simulink subsystem "shaping"  (R2024b)
settings: Solver=VariableStepAuto  StartTime=0.0  StopTime=10.0  RelTol=1e-3
model mask{c_srrc_coef=0, c_inter_1_coef=0, c_inter_2_coef=0}
  mask prompts: c_srrc_coef "Interpolator SRRC  stage coefficients"; c_inter_1_coef "Interpolator 1 coefficients"; c_inter_2_coef "Interpolator 2 coefficients"
values from neighbouring files (symbols this model uses):
  c_srrc_coef = jsonData.shaping.c_srrc_coef    [seq.m]
libraries: hdlsllib x10, dsphdlfiltering2 x3
settings Model: Creator=usradmin  LastModifiedBy=jose.sanchez
settings RTWCC: GPUComputeCapability=3.5

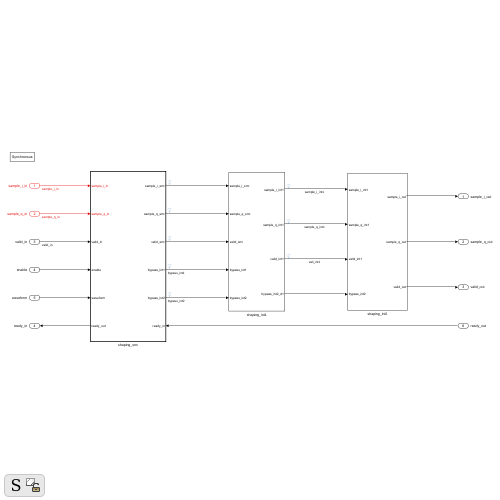
[thumbnail: Simulink's stored preview of the top-level diagram]
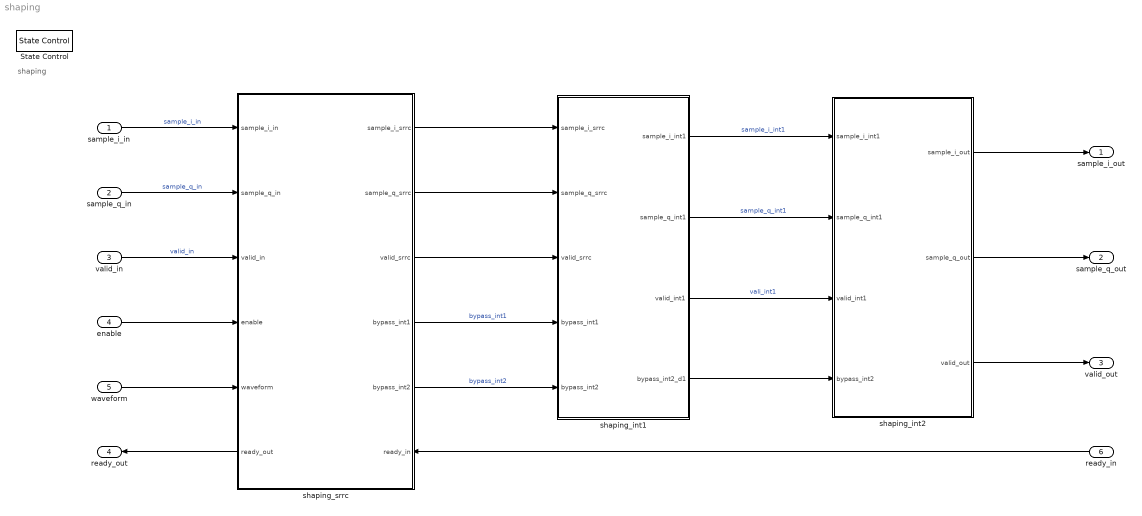
== system shaping ==
  note: shaping
  sample_i_in : Inport  OutDataTypeStr=fixdt(1,16,15)
  sample_q_in : Inport  Port=2  OutDataTypeStr=fixdt(1,16,15)
  valid_in : Inport  Port=3  OutDataTypeStr=boolean
  enable : Inport  Port=4  OutDataTypeStr=boolean
  waveform : Inport  Port=5  OutMin=[0]  OutMax=[3]  OutDataTypeStr=fixdt(0,2)
  ready_in : Inport  Port=6  OutDataTypeStr=boolean
  State Control : StateControl  StateControl=Synchronous
  shaping_int1 : Subsystem
  shaping_int2 : Subsystem
  shaping_srrc : Subsystem
      settings: PortSchema="{\"entries\":[{\"content\":{\"sides\":[{\"content\":{\"connectorIds\":[\"In1\",\"In2\",\"In3\",\"In4\",\"In5\",\"Out6\"]},\"type\":\"ConnectorPlacement.EquallySpacedRectSide\",\"uuid\":\"d1664757-8441-4e5c-b538-f30b5bedf7ee\"},{\"content\":{\"connectorIds\":[\"Out1\",\"Out2\",\"Out3\",\"Out4\",\"Out5\",\"In6\"],\"side\":\"RIGHT\"},\"type\":\"ConnectorPlacement.EquallySpacedRectSide\",\"uuid\":\"660e1ba2-a444-4ece-b784-c0538aecc110\"},{\"content\":{\"side\":\"TOP\"},\"type\":\"ConnectorPlacement.EquallySpacedRectSide\",\"uuid\":\"adc6c3d6-bacf-46d3-9822-3cabe58d745e\"}]},\"type\":\"ConnectorPlacement.EquallySpacedConnector\",\"uuid\":\"1ec29908-4970-4c2d-ab54-8f6747339545\"}],\"packageUris\":[\"http://schema.mathworks.com/mf0/Connector/R2020b\"],\"version\":\"1.0\"}"
  sample_i_out : Outport  OutDataTypeStr=fixdt(1,16,14)
  sample_q_out : Outport  Port=2  OutDataTypeStr=fixdt(1,16,14)
  valid_out : Outport  Port=3  OutDataTypeStr=boolean
  ready_out : Outport  Port=4  OutDataTypeStr=boolean
  wires:
  sample_i_in/1 -> shaping_srrc/1(sample_i_in)  "sample_i_in"
  sample_q_in/1 -> shaping_srrc/2(sample_q_in)  "sample_q_in"
  valid_in/1 -> shaping_srrc/3(valid_in)  "valid_in"
  shaping_srrc/6(ready_out) -> ready_out/1
  enable/1 -> shaping_srrc/4(enable)
  waveform/1 -> shaping_srrc/5(waveform)
  shaping_srrc/1(sample_i_srrc) -> shaping_int1/1(sample_i_srrc)
  shaping_srrc/2(sample_q_srrc) -> shaping_int1/2(sample_q_srrc)
  shaping_srrc/3(valid_srrc) -> shaping_int1/3(valid_srrc)
  shaping_srrc/4(bypass_int1) -> shaping_int1/4(bypass_int1)  "bypass_int1"
  shaping_int1/1(sample_i_int1) -> shaping_int2/1(sample_i_int1)  "sample_i_int1"
  shaping_int1/2(sample_q_int1) -> shaping_int2/2(sample_q_int1)  "sample_q_int1"
  shaping_int1/3(valid_int1) -> shaping_int2/3(valid_int1)  "vali_int1"
  shaping_int2/1(sample_i_out) -> sample_i_out/1
  shaping_int2/2(sample_q_out) -> sample_q_out/1
  shaping_int2/3(valid_out) -> valid_out/1
  ready_in/1 -> shaping_srrc/6(ready_in)
  shaping_srrc/5(bypass_int2) -> shaping_int1/5(bypass_int2)  "bypass_int2"
  shaping_int1/4(bypass_int2_d1) -> shaping_int2/4(bypass_int2)

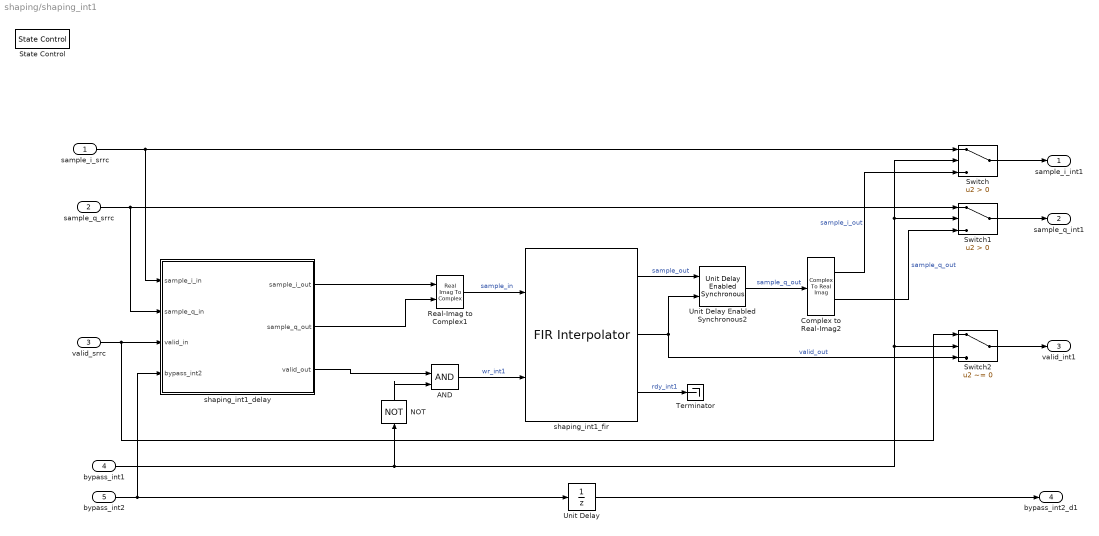
== system shaping/shaping_int1 ==
  sample_i_srrc : Inport
  sample_q_srrc : Inport  Port=2
  valid_srrc : Inport  Port=3
  bypass_int1 : Inport  Port=4
  bypass_int2 : Inport  Port=5
  AND : Logic  IconShape=distinctive  AllPortsSameDT=off  OutDataTypeStr=boolean
  Complex to Real-Imag2 : ComplexToRealImag
  NOT : Logic  Operator=NOT  IconShape=distinctive  AllPortsSameDT=off  OutDataTypeStr=boolean
  Real-Imag to Complex1 : RealImagToComplex
  State Control : StateControl  StateControl=Synchronous
  Switch : Switch  Criteria=u2 > Threshold  SaturateOnIntegerOverflow=off  InputSameDT=off
  Switch1 : Switch  Criteria=u2 > Threshold  SaturateOnIntegerOverflow=off  InputSameDT=off
  Switch2 : Switch  Criteria=u2 ~= 0  SaturateOnIntegerOverflow=off  InputSameDT=off
  Terminator : Terminator
  Unit Delay : UnitDelay  SampleTime=-1  HasFrameUpgradeWarning=on
  Unit Delay Enabled Synchronous2 : hdlsllib/Discrete/Unit Delay Enabled Synchronous  InitialCondition=0.0  SampleTime=-1
  shaping_int1_delay : Subsystem
  shaping_int1_fir : dsphdlfiltering2/FIR Interpolator  Numerator=c_inter_1_coef  FilterStructure=Direct form systolic  InterpolationFactor=2  NumCycles=2  OptimizeSymmCoeff=on  SimulateUsing=Code generation  roundingMode=Floor  overflowMode=off  CoefficientsDataTypeStr=fixdt(1,16,15)  OutputDataTypeStr=fixdt(1,16,14)  ResetInputPort=off  HDLGlobalReset=on
  sample_i_int1 : Outport
  sample_q_int1 : Outport  Port=2
  valid_int1 : Outport  Port=3
  bypass_int2_d1 : Outport  Port=4
  wires:
  Unit Delay/1 -> bypass_int2_d1/1
  bypass_int2/1 -> Unit Delay/1, shaping_int1_delay/4(bypass_int2)
  valid_srrc/1 -> shaping_int1_delay/3(valid_in), Switch2/1
  sample_q_srrc/1 -> shaping_int1_delay/2(sample_q_in), Switch1/1
  sample_i_srrc/1 -> Switch/1, shaping_int1_delay/1(sample_i_in)
  shaping_int1_fir/3 -> Terminator/1  "rdy_int1"
  Switch2/1 -> valid_int1/1
  Real-Imag to Complex1/1 -> shaping_int1_fir/1  "sample_in"
  shaping_int1_delay/2(sample_q_out) -> Real-Imag to Complex1/2
  bypass_int1/1 -> NOT/1, Switch2/2, Switch1/2, Switch/2
  shaping_int1_delay/3(valid_out) -> AND/1
  Switch/1 -> sample_i_int1/1
  AND/1 -> shaping_int1_fir/2  "wr_int1"
  Complex to Real-Imag2/2 -> Switch1/3  "sample_q_out"
  Switch1/1 -> sample_q_int1/1
  shaping_int1_delay/1(sample_i_out) -> Real-Imag to Complex1/1
  Unit Delay Enabled Synchronous2/1 -> Complex to Real-Imag2/1  "sample_q_out"
  shaping_int1_fir/2 -> Unit Delay Enabled Synchronous2/2, Switch2/3  "valid_out"
  shaping_int1_fir/1 -> Unit Delay Enabled Synchronous2/1  "sample_out"
  NOT/1 -> AND/2
  Complex to Real-Imag2/1 -> Switch/3  "sample_i_out"

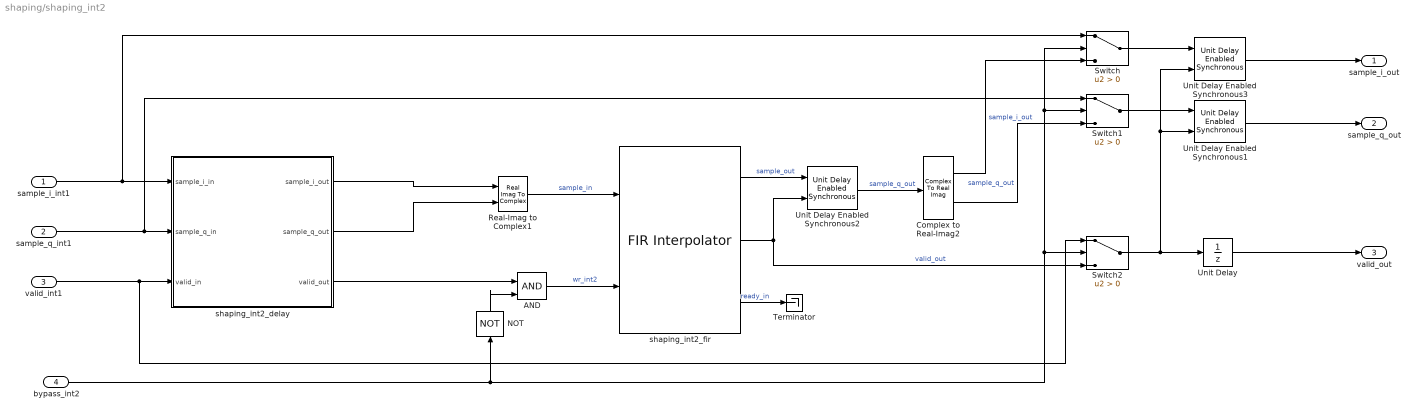
== system shaping/shaping_int2 ==
  sample_i_int1 : Inport
  sample_q_int1 : Inport  Port=2
  valid_int1 : Inport  Port=3
  bypass_int2 : Inport  Port=4
  AND : Logic  IconShape=distinctive  AllPortsSameDT=off  OutDataTypeStr=boolean
  Complex to Real-Imag2 : ComplexToRealImag
  NOT : Logic  Operator=NOT  IconShape=distinctive  AllPortsSameDT=off  OutDataTypeStr=boolean
  Real-Imag to Complex1 : RealImagToComplex
  Switch : Switch  Criteria=u2 > Threshold  SaturateOnIntegerOverflow=off  InputSameDT=off
  Switch1 : Switch  Criteria=u2 > Threshold  SaturateOnIntegerOverflow=off  InputSameDT=off
  Switch2 : Switch  Criteria=u2 > Threshold  SaturateOnIntegerOverflow=off  InputSameDT=off
  Terminator : Terminator
  Unit Delay : UnitDelay  SampleTime=-1  HasFrameUpgradeWarning=on
  Unit Delay Enabled Synchronous1 : hdlsllib/Discrete/Unit Delay Enabled Synchronous  InitialCondition=0.0  SampleTime=-1
  Unit Delay Enabled Synchronous2 : hdlsllib/Discrete/Unit Delay Enabled Synchronous  InitialCondition=0.0  SampleTime=-1
  Unit Delay Enabled Synchronous3 : hdlsllib/Discrete/Unit Delay Enabled Synchronous  InitialCondition=0.0  SampleTime=-1
  shaping_int2_delay : Subsystem
  shaping_int2_fir : dsphdlfiltering2/FIR Interpolator  Numerator=c_inter_2_coef  FilterStructure=Direct form systolic  InterpolationFactor=2  NumCycles=2  OptimizeSymmCoeff=on  SimulateUsing=Code generation  roundingMode=Floor  overflowMode=off  CoefficientsDataTypeStr=fixdt(1,16,15)  OutputDataTypeStr=fixdt(1,16,14)  ResetInputPort=off  HDLGlobalReset=on
  sample_i_out : Outport
  sample_q_out : Outport  Port=2
  valid_out : Outport  Port=3
  wires:
  valid_int1/1 -> shaping_int2_delay/3(valid_in), Switch2/1
  sample_q_int1/1 -> shaping_int2_delay/2(sample_q_in), Switch1/1
  sample_i_int1/1 -> shaping_int2_delay/1(sample_i_in), Switch/1
  Unit Delay/1 -> valid_out/1
  Switch/1 -> Unit Delay Enabled Synchronous3/1
  Switch1/1 -> Unit Delay Enabled Synchronous1/1
  Complex to Real-Imag2/1 -> Switch/3  "sample_i_out"
  NOT/1 -> AND/2
  shaping_int2_fir/1 -> Unit Delay Enabled Synchronous2/1  "sample_out"
  shaping_int2_fir/2 -> Unit Delay Enabled Synchronous2/2, Switch2/3  "valid_out"
  Unit Delay Enabled Synchronous2/1 -> Complex to Real-Imag2/1  "sample_q_out"
  shaping_int2_delay/1(sample_i_out) -> Real-Imag to Complex1/1
  Unit Delay Enabled Synchronous1/1 -> sample_q_out/1
  shaping_int2_fir/3 -> Terminator/1  "ready_in"
  Complex to Real-Imag2/2 -> Switch1/3  "sample_q_out"
  AND/1 -> shaping_int2_fir/2  "wr_int2"
  Unit Delay Enabled Synchronous3/1 -> sample_i_out/1
  shaping_int2_delay/3(valid_out) -> AND/1
  bypass_int2/1 -> NOT/1, Switch1/2, Switch/2, Switch2/2
  shaping_int2_delay/2(sample_q_out) -> Real-Imag to Complex1/2
  Real-Imag to Complex1/1 -> shaping_int2_fir/1  "sample_in"
  Switch2/1 -> Unit Delay/1, Unit Delay Enabled Synchronous3/2, Unit Delay Enabled Synchronous1/2

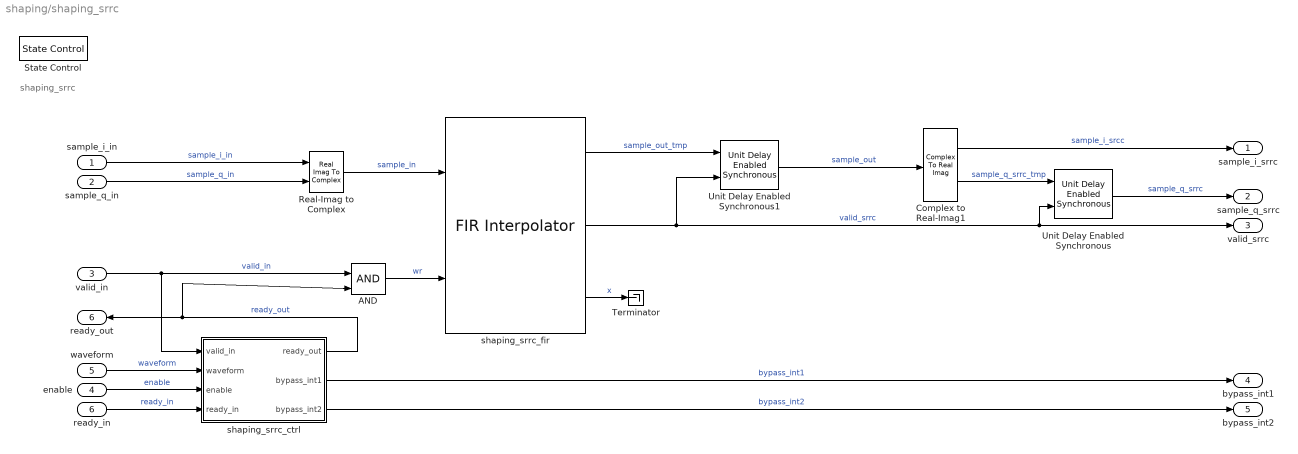
== system shaping/shaping_srrc ==
  note: shaping_srrc
  sample_i_in : Inport  OutDataTypeStr=fixdt(1,16,15)
  sample_q_in : Inport  Port=2  OutDataTypeStr=fixdt(1,16,15)
  valid_in : Inport  Port=3  OutDataTypeStr=boolean
  enable : Inport  Port=4  OutDataTypeStr=boolean
  waveform : Inport  Port=5  OutMin=[0]  OutMax=[3]  OutDataTypeStr=fixdt(0,2)
  ready_in : Inport  Port=6  OutDataTypeStr=boolean
  AND : Logic  IconShape=distinctive  AllPortsSameDT=off  OutDataTypeStr=boolean
  Complex to Real-Imag1 : ComplexToRealImag
  Real-Imag to Complex : RealImagToComplex
  State Control : StateControl  StateControl=Synchronous
  Terminator : Terminator
  Unit Delay Enabled Synchronous : hdlsllib/Discrete/Unit Delay Enabled Synchronous  InitialCondition=0.0  SampleTime=-1
  Unit Delay Enabled Synchronous1 : hdlsllib/Discrete/Unit Delay Enabled Synchronous  InitialCondition=0.0  SampleTime=-1
  shaping_srrc_ctrl : MATLAB Function  TreatAsAtomicUnit=on
  shaping_srrc_fir : dsphdlfiltering2/FIR Interpolator  Numerator=c_srrc_coef  FilterStructure=Direct form systolic  InterpolationFactor=2  NumCycles=2  OptimizeSymmCoeff=on  SimulateUsing=Code generation  roundingMode=Floor  overflowMode=off  CoefficientsDataTypeStr=fixdt(1,16,15)  OutputDataTypeStr=fixdt(1,16,14)  ResetInputPort=off  HDLGlobalReset=on
  sample_i_srrc : Outport
  sample_q_srrc : Outport  Port=2
  valid_srrc : Outport  Port=3  OutDataTypeStr=boolean
  bypass_int1 : Outport  Port=4  OutDataTypeStr=boolean
  bypass_int2 : Outport  Port=5  OutDataTypeStr=boolean
  ready_out : Outport  Port=6  OutDataTypeStr=boolean
  wires:
  ready_in/1 -> shaping_srrc_ctrl/4(ready_in)  "ready_in"
  shaping_srrc_fir/3 -> Terminator/1  "x"
  shaping_srrc_ctrl/3(bypass_int2) -> bypass_int2/1  "bypass_int2"
  shaping_srrc_ctrl/2(bypass_int1) -> bypass_int1/1  "bypass_int1"
  Unit Delay Enabled Synchronous/1 -> sample_q_srrc/1  "sample_q_srrc"
  valid_in/1 -> shaping_srrc_ctrl/1(valid_in), AND/1  "valid_in"
  sample_i_in/1 -> Real-Imag to Complex/1  "sample_i_in"
  enable/1 -> shaping_srrc_ctrl/3(enable)  "enable"
  shaping_srrc_ctrl/1(ready_out) -> ready_out/1, AND/2  "ready_out"
  Real-Imag to Complex/1 -> shaping_srrc_fir/1  "sample_in"
  shaping_srrc_fir/2 -> Unit Delay Enabled Synchronous1/2, Unit Delay Enabled Synchronous/2, valid_srrc/1  "valid_srrc"
  AND/1 -> shaping_srrc_fir/2  "wr"
  Complex to Real-Imag1/1 -> sample_i_srrc/1  "sample_i_srcc"
  waveform/1 -> shaping_srrc_ctrl/2(waveform)  "waveform"
  Complex to Real-Imag1/2 -> Unit Delay Enabled Synchronous/1  "sample_q_srrc_tmp"
  shaping_srrc_fir/1 -> Unit Delay Enabled Synchronous1/1  "sample_out_tmp"
  sample_q_in/1 -> Real-Imag to Complex/2  "sample_q_in"
  Unit Delay Enabled Synchronous1/1 -> Complex to Real-Imag1/1  "sample_out"

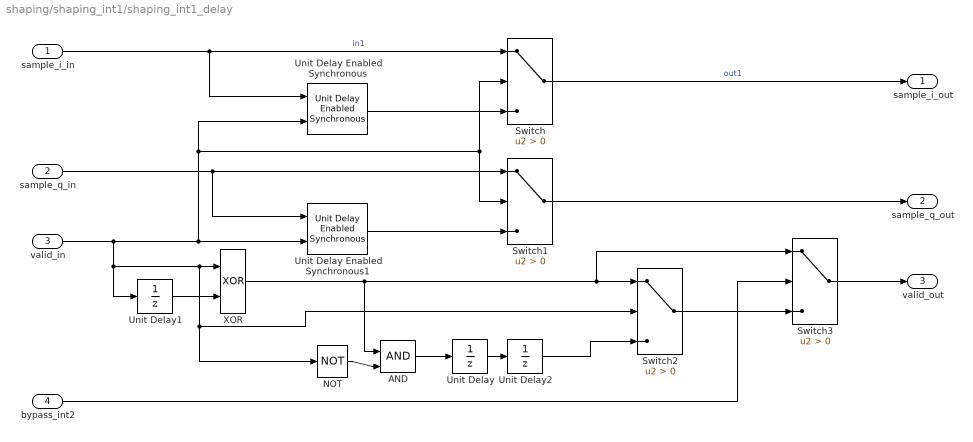
== system shaping/shaping_int1/shaping_int1_delay ==
  sample_i_in : Inport
  sample_q_in : Inport  Port=2
  valid_in : Inport  Port=3
  bypass_int2 : Inport  Port=4
  AND : Logic  IconShape=distinctive  AllPortsSameDT=off  OutDataTypeStr=boolean
  NOT : Logic  Operator=NOT  IconShape=distinctive  AllPortsSameDT=off  OutDataTypeStr=boolean
  Switch{,1..3} (4 alike) : Switch  Criteria=u2 > Threshold  SaturateOnIntegerOverflow=off  InputSameDT=off
  Unit Delay : UnitDelay  SampleTime=-1  HasFrameUpgradeWarning=on
  Unit Delay Enabled Synchronous : hdlsllib/Discrete/Unit Delay Enabled Synchronous  InitialCondition=0  SampleTime=-1
  Unit Delay Enabled Synchronous1 : hdlsllib/Discrete/Unit Delay Enabled Synchronous  InitialCondition=0  SampleTime=-1
  Unit Delay1 : UnitDelay  SampleTime=-1  HasFrameUpgradeWarning=on
  Unit Delay2 : UnitDelay  SampleTime=-1  HasFrameUpgradeWarning=on
  XOR : Logic  Operator=XOR  IconShape=distinctive  AllPortsSameDT=off  OutDataTypeStr=boolean
  sample_i_out : Outport  VectorParamsAs1DForOutWhenUnconnected=off
  sample_q_out : Outport  Port=2  VectorParamsAs1DForOutWhenUnconnected=off
  valid_out : Outport  Port=3  VectorParamsAs1DForOutWhenUnconnected=off
  wires:
  Unit Delay1/1 -> XOR/2
  Switch/1 -> sample_i_out/1  "out1"
  AND/1 -> Unit Delay/1
  Switch1/1 -> sample_q_out/1
  sample_q_in/1 -> Unit Delay Enabled Synchronous1/1, Switch1/1
  sample_i_in/1 -> Unit Delay Enabled Synchronous/1, Switch/1  "in1"
  Unit Delay2/1 -> Switch2/3
  NOT/1 -> AND/2
  Unit Delay/1 -> Unit Delay2/1
  Unit Delay Enabled Synchronous1/1 -> Switch1/3
  Switch2/1 -> Switch3/3
  XOR/1 -> AND/1, Switch2/1, Switch3/1
  Unit Delay Enabled Synchronous/1 -> Switch/3
  valid_in/1 -> Unit Delay Enabled Synchronous1/2, Switch/2, Switch1/2, Unit Delay Enabled Synchronous/2, XOR/1, NOT/1, Switch2/2, Unit Delay1/1
  bypass_int2/1 -> Switch3/2
  Switch3/1 -> valid_out/1

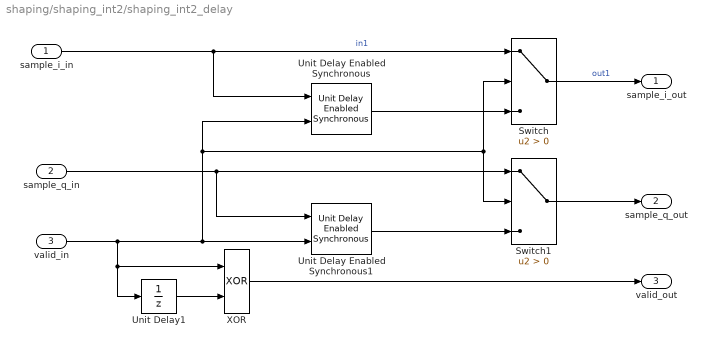
== system shaping/shaping_int2/shaping_int2_delay ==
  sample_i_in : Inport
  sample_q_in : Inport  Port=2
  valid_in : Inport  Port=3
  Switch : Switch  Criteria=u2 > Threshold  SaturateOnIntegerOverflow=off  InputSameDT=off
  Switch1 : Switch  Criteria=u2 > Threshold  SaturateOnIntegerOverflow=off  InputSameDT=off
  Unit Delay Enabled Synchronous : hdlsllib/Discrete/Unit Delay Enabled Synchronous  InitialCondition=0  SampleTime=-1
  Unit Delay Enabled Synchronous1 : hdlsllib/Discrete/Unit Delay Enabled Synchronous  InitialCondition=0  SampleTime=-1
  Unit Delay1 : UnitDelay  SampleTime=-1  HasFrameUpgradeWarning=on
  XOR : Logic  Operator=XOR  IconShape=distinctive  AllPortsSameDT=off  OutDataTypeStr=boolean
  sample_i_out : Outport  VectorParamsAs1DForOutWhenUnconnected=off
  sample_q_out : Outport  Port=2  VectorParamsAs1DForOutWhenUnconnected=off
  valid_out : Outport  Port=3  VectorParamsAs1DForOutWhenUnconnected=off
  wires:
  XOR/1 -> valid_out/1
  Unit Delay1/1 -> XOR/2
  Unit Delay Enabled Synchronous1/1 -> Switch1/3
  valid_in/1 -> Unit Delay Enabled Synchronous1/2, Switch/2, Switch1/2, Unit Delay Enabled Synchronous/2, XOR/1, Unit Delay1/1
  Switch1/1 -> sample_q_out/1
  Switch/1 -> sample_i_out/1  "out1"
  Unit Delay Enabled Synchronous/1 -> Switch/3
  sample_i_in/1 -> Unit Delay Enabled Synchronous/1, Switch/1  "in1"
  sample_q_in/1 -> Unit Delay Enabled Synchronous1/1, Switch1/1

== matlab function shaping/shaping_srrc/shaping_srrc_ctrl ==
  data: valid_in input; ready_out output; waveform input; enable input; bypass_int1 output; bypass_int2 output; ready_in input
function [ready_out, bypass_int1, bypass_int2] = fcn(valid_in, waveform, enable, ready_in)

    % ---------------------------------------------------------------------
    % TYPES DEFINITION
    % ---------------------------------------------------------------------
    std_2 = numerictype(0,2,0);
    std_3 = numerictype(0,3,0);

    % ---------------------------------------------------------------------
    % REGISTERS DEFINITION
    % ---------------------------------------------------------------------
    persistent cnt_reg
    if isempty(cnt_reg)
        cnt_reg = fi(1, std_3);
    end

    % ---------------------------------------------------------------------
    % ASIGNATION DEFINITION
    % ---------------------------------------------------------------------

    % ---------------------------------------------------------------------
    % PROCESS DEFINITION
    % ---------------------------------------------------------------------
    % Select the filter in waveform funcion
    % waveform = 3 -> SRCC
    % waveform = 2 -> SRRC + INT1
    % Waveform = 1 -> SRRC + INT1 + INT2
    %
    if (waveform == fi(3, std_2))
        bypass_int1 = true;
        bypass_int2 = true;
    elseif (waveform == fi(2, std_2))
        bypass_int1 = false;
        bypass_int2 = true;
    else
        bypass_int1 = false;
        bypass_int2 = false;
    end

    % Requst data from before module in waveform function
    % waveform = 3 -> 1 data each 2 clock cycles
    % waveform = 2 -> 1 data each 4 clock cycles
    % waveform = 1 -> 1 data each 8 clock cycles
    %
    if (waveform == fi(3, std_2) && (cnt_reg == fi(0, std_3) || cnt_reg == fi(2, std_3) || cnt_reg == fi(4, std_3) || cnt_reg == fi(6, std_3))) || ...
       (waveform == fi(2, std_2) && (cnt_reg == fi(0, std_3) || cnt_reg == fi(4, std_3))) || ...
       (waveform == fi(1, std_2) && cnt_reg == fi(0, std_3))

        ready_out = ready_in;
    else
        ready_out = false;
    end

    if (not(enable))
        cnt_reg = fi(1, std_3);
    elseif (valid_in)
        if (cnt_reg == fi(7, std_3) && ready_in)
           cnt_reg = fi(0, std_3); 
        else
            if (cnt_reg < fi(7, std_3))
                inc = cnt_reg + 1;
                cnt_reg = fi(inc, std_3);
            end 
        end
    end
    % ---------------------------------------------------------------------
    % END
    % ---------------------------------------------------------------------
